simulink model "complete"  (R2019b)
settings: Solver=VariableStepAuto  StartTime=0.0  StopTime=200  RelTol=1e-3
values from neighbouring files (symbols this model uses):
  battery =     [battery.mat]    (also in batteryModel_Sfcn.m = block.DialogPrm(1).Data)
  controllers =     [controllers.mat]
  IC = block.DialogPrm(2).Data    [Dynamics.m]    (also in IC_HoverAt10ftOcto.mat = ; IC_HoverAt10ftOctoWithMotorControl.mat = )
  Motor =     [DJI4114_400kv_BLDC_Motor.mat]
  octomodel =     [octoModel.mat]
undefined symbols (not defined in the file or in its folder): DiscIntNeverNeededParam
libraries: simulink x1
(part 2 of 2)

== matlab function complete/Motors/DC Motor 2/Mechanical part/speed - torque load relationship we will not consider for now/Propeller model  ==
  data: torque output; rpm input; thrust output
function [torque,thrust] = fcn(rpm)
% angular_velocity in rpm
if rpm>2000
    see=1;
end
%coefficient of thrust, empirically derived
coef_t = 0.0524;
%thrust = coef_t * density of air * velocity^2 * propeller diameter (m) ^4
%velocity in rev/sec, where  1 rev/sec = 1 rpm/60
thrust = coef_t*1.225*(rpm/60)^2*.381^4; % 15 inches ~ 0.381 m
% empirically derived
torque = (1.065e-08)*rpm^2 + (-3.45e-06)*rpm + (0.0064);

end

== matlab function complete/Motors/DC Motor 3/Mechanical part/speed - torque load relationship we will not consider for now/Propeller model  ==
  data: torque output; rpm input; thrust output
function [torque,thrust] = fcn(rpm)
% angular_velocity in rpm
if rpm>2000
    see=1;
end
%coefficient of thrust, empirically derived
coef_t = 0.0524;
%thrust = coef_t * density of air * velocity^2 * propeller diameter (m) ^4
%velocity in rev/sec, where  1 rev/sec = 1 rpm/60
thrust = coef_t*1.225*(rpm/60)^2*.381^4; % 15 inches ~ 0.381 m
% empirically derived
torque = (1.065e-08)*rpm^2 + (-3.45e-06)*rpm + (0.0064);

end

== matlab function complete/Motors/DC Motor 4/Mechanical part/speed - torque load relationship we will not consider for now/Propeller model  ==
  data: torque output; rpm input; thrust output
function [torque,thrust] = fcn(rpm)
% angular_velocity in rpm
if rpm>2000
    see=1;
end
%coefficient of thrust, empirically derived
coef_t = 0.0524;
%thrust = coef_t * density of air * velocity^2 * propeller diameter (m) ^4
%velocity in rev/sec, where  1 rev/sec = 1 rpm/60
thrust = coef_t*1.225*(rpm/60)^2*.381^4; % 15 inches ~ 0.381 m
% empirically derived
torque = (1.065e-08)*rpm^2 + (-3.45e-06)*rpm + (0.0064);

end

== matlab function complete/Motors/DC Motor 5/Mechanical part/speed - torque load relationship we will not consider for now/Propeller model  ==
  data: torque output; rpm input; thrust output
function [torque,thrust] = fcn(rpm)
% angular_velocity in rpm
if rpm>2000
    see=1;
end
%coefficient of thrust, empirically derived
coef_t = 0.0524;
%thrust = coef_t * density of air * velocity^2 * propeller diameter (m) ^4
%velocity in rev/sec, where  1 rev/sec = 1 rpm/60
thrust = coef_t*1.225*(rpm/60)^2*.381^4; % 15 inches ~ 0.381 m
% empirically derived
torque = (1.065e-08)*rpm^2 + (-3.45e-06)*rpm + (0.0064);

end

== matlab function complete/Motors/DC Motor 6/Mechanical part/speed - torque load relationship we will not consider for now/Propeller model  ==
  data: torque output; rpm input; thrust output
function [torque,thrust] = fcn(rpm)
% angular_velocity in rpm
if rpm>2000
    see=1;
end
%coefficient of thrust, empirically derived
coef_t = 0.0524;
%thrust = coef_t * density of air * velocity^2 * propeller diameter (m) ^4
%velocity in rev/sec, where  1 rev/sec = 1 rpm/60
thrust = coef_t*1.225*(rpm/60)^2*.381^4; % 15 inches ~ 0.381 m
% empirically derived
torque = (1.065e-08)*rpm^2 + (-3.45e-06)*rpm + (0.0064);

end

== matlab function complete/Motors/DC Motor 7/Mechanical part/speed - torque load relationship we will not consider for now/Propeller model  ==
  data: torque output; rpm input; thrust output
function [torque,thrust] = fcn(rpm)
% angular_velocity in rpm
if rpm>2000
    see=1;
end
%coefficient of thrust, empirically derived
coef_t = 0.0524;
%thrust = coef_t * density of air * velocity^2 * propeller diameter (m) ^4
%velocity in rev/sec, where  1 rev/sec = 1 rpm/60
thrust = coef_t*1.225*(rpm/60)^2*.381^4; % 15 inches ~ 0.381 m
% empirically derived
torque = (1.065e-08)*rpm^2 + (-3.45e-06)*rpm + (0.0064);

end

== matlab function complete/Control allocation ==
  data: Fx input; wref1 output; Fy input; Fz input; Troll input; Tpitch input; Tyaw input; wref2 output; wref3 output; wref4 output; wref5 output; wref6 output; wref7 output; wref8 output
function [wref1,wref2,wref3,wref4,wref5,wref6,wref7,wref8] = fcn(Fx,Fy,Fz,Troll,Tpitch,Tyaw)

%% parameters required
% load('params/octoModel.mat');
gamma=3;%octomodel.tiltmotorangle;
alpha=45;%octomodel.separationmotorangle;
dl=0.45;%octomodel.dl;
constant=(1/sqrt(2));
ds=0.35;%octomodel.ds;
ct=3.4262e-05;%octomodel.ct*(60/(2*pi))^2 -> in octomodel is for rpm, here I need it in rad/s;
cq=9.3846e-07;%octomodel.cq*(60/(2*pi))^2 -> in octomodel is for rpm, here I need it in rad/s;

%% rotation matrices because of 3 degrees tilted angle

E_m_b = [0 -sin(alpha)*sin(gamma) sin(gamma) -cos(alpha)*sin(gamma) 0 sin(alpha)*sin(gamma) -sin(gamma) cos(alpha)*sin(gamma);
         -sin(gamma)  cos(alpha)*sin(gamma) 0 -sin(alpha)*sin(gamma) sin(gamma) -cos(alpha)*sin(gamma) 0 sin(alpha)*sin(gamma);
         -cos(gamma) -cos(gamma) -cos(gamma) -cos(gamma) -cos(gamma) -cos(gamma) -cos(gamma) -cos(gamma)];

R_m=[dl 0 0; ...
    constant*ds constant*ds 0; ...
    0 dl 0; ...
    -constant*ds constant*ds 0; ...
    -dl 0 0; ...
    -constant*ds -constant*ds 0; ...
    0 -dl 0; ...
    constant*ds -constant*ds 0]';

%% first form delta_b matrix
%a vectors
a=zeros(3,8);
for i=1:8
    e_i_b=E_m_b(:,i);
    a(:,i)=(ct).*e_i_b;
end

%b vectors
b=zeros(3,8);
for i=1:8
    e_i_b=E_m_b(:,i);
    r_m=R_m(:,i);
    b(:,i)=cross( r_m,(ct).*e_i_b ) + ((-1)^(i+1)*(cq)).*e_i_b;    
end

%form matrix
delta_b=[a;b];

%find pseudo-inverse
delta_binv = pinv(delta_b);

%% calculate required w_ref
Forces=[Fx,Fy,Fz];
Torques=[Troll,Tpitch,Tyaw];
if Troll>0
    see=1;
end
input=[Forces,Torques]';
wref=delta_binv*input;
%check if complex
if(isreal(wref(2)) )
    see=1;
end

if length(find(wref<0))>0
    pos=find(wref<0);
    wref(pos)=0;
end
wref=sqrt(wref);

% %angular velocity in rad/s
% wref1=wref(1);
% wref2=wref(2);
% wref3=wref(3);
% wref4=wref(4);
% wref5=wref(5);
% wref6=wref(6);
% wref7=wref(7);
% wref8=wref(8);

%angular velocity in rpm
% wref1=wref(1)*(60/(2*pi));
% wref2=wref(2)*(60/(2*pi));
% wref3=wref(3)*(60/(2*pi));
% wref4=wref(4)*(60/(2*pi));
% wref5=wref(5)*(60/(2*pi));
% wref6=wref(6)*(60/(2*pi));
% wref7=wref(7)*(60/(2*pi));
% wref8=wref(8)*(60/(2*pi));

%% now convert to voltage in the range 0-22V
% divide=36.17; %true is 36.37
% multiply=0.0238; %for 8800 rpm nominal 
multiply=0.02762; %for 6783 rpm considering torque load 
wref1=wref(1)*multiply;
wref2=wref(2)*multiply;
wref3=wref(3)*multiply;
wref4=wref(4)*multiply;
wref5=wref(5)*multiply;
wref6=wref(6)*multiply;
wref7=wref(7)*multiply;
wref8=wref(8)*multiply;

see=1;

end

== matlab function complete/Battery cell/OCV from SOC ==
  data: soc input; ocv output; soc_ocv input
function ocv = getOCVplain(soc, soc_ocv)
    if soc < 0.0
        soc = 0;
    elseif soc > 1.0
        soc = 1.0;
    end
    
    idx = ceil(soc*100);
    
    if idx > 101
        idx = 101;
    elseif idx < 1
        idx = 1;
    end
    ocv = soc_ocv(idx);
end

== matlab function complete/Motors/DC Motor /Mechanical part/speed - torque load relationship we will not consider for now/Propeller model  ==
  data: torque output; rpm input; thrust output
function [torque,thrust] = fcn(rpm)
% angular_velocity in rpm
if rpm>2000
    see=1;
end
%coefficient of thrust, empirically derived
coef_t = 0.0524;
%thrust = coef_t * density of air * velocity^2 * propeller diameter (m) ^4
%velocity in rev/sec, where  1 rev/sec = 1 rpm/60
thrust = coef_t*1.225*(rpm/60)^2*.381^4; % 15 inches ~ 0.381 m
% empirically derived
torque = (1.065e-08)*rpm^2 + (-3.45e-06)*rpm + (0.0064);

end
